simulink subsystem "airframeWeight"  (R2023b)
settings: Solver=VariableStepAuto  StartTime=0.0  StopTime=10.0  RelTol=1e-3
undefined symbols (not defined in the file): g, mass
libraries: sharedtransform x1
settings Model: Creator=Victor  LastModifiedBy=Victor

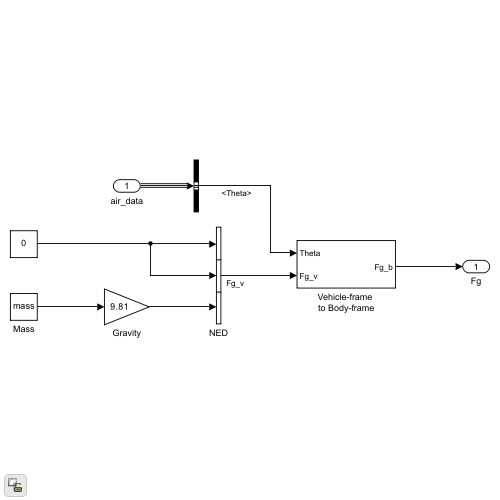
[thumbnail: Simulink's stored preview of the top-level diagram]
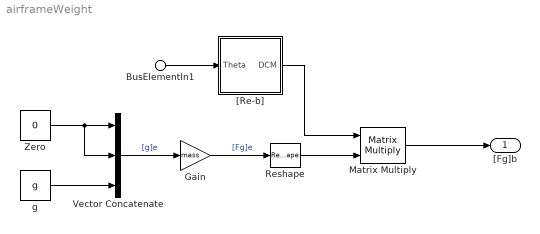
== system airframeWeight ==
  BusElementIn1 : Inport  PortName=uavBus  Element=stateBus.[Theta]b
  Gain : Gain  Gain=mass
  Matrix Multiply : Product  Multiplication=Matrix(*)
  Reshape : Reshape  OutputDimensionality=Column vector (2-D)
  Vector Concatenate : Concatenate  NumInputs=3
  Zero : Constant  Value=0  OutDataTypeStr=Inherit: Inherit via back propagation
  "[Re-b]" : Subsystem
  g : Constant  Value=g
  "[Fg]b" : Outport
  wires:
  Zero/1 -> Vector Concatenate/1, Vector Concatenate/2
  g/1 -> Vector Concatenate/3
  Vector Concatenate/1 -> Gain/1  "[g]e"
  Reshape/1 -> Matrix Multiply/2
  Matrix Multiply/1 -> "[Fg]b"/1
  BusElementIn1/1 -> "[Re-b]"/1(Theta)
  "[Re-b]"/1(DCM) -> Matrix Multiply/1
  Gain/1 -> Reshape/1  "[Fg]e"

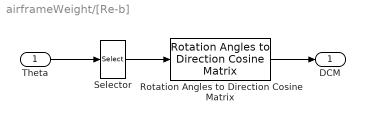
== system airframeWeight/[Re-b] ==
  Theta : Inport
  Rotation Angles to Direction Cosine Matrix : sharedtransform/Rotation Angles to Direction Cosine Matrix  rotationOrder=ZYX  aMode=aMode
  Selector : Selector  InputPortWidth=3  IndexOptions=Index vector (dialog)  Indices=[3 2 1]  OutputSizes=1
  DCM : Outport  OutDataTypeStr=double  VectorParamsAs1DForOutWhenUnconnected=off
  wires:
  Selector/1 -> Rotation Angles to Direction Cosine Matrix/1
  Theta/1 -> Selector/1
  Rotation Angles to Direction Cosine Matrix/1 -> DCM/1
